simulink model "Problem_8_LIFT"  (R2020b)
settings: Solver=VariableStepAuto  StartTime=0.0  StopTime=10.0  RelTol=1e-3
settings Model: PacingRate=0.450000  Creator=Manoj  LastModifiedBy=Windows 10

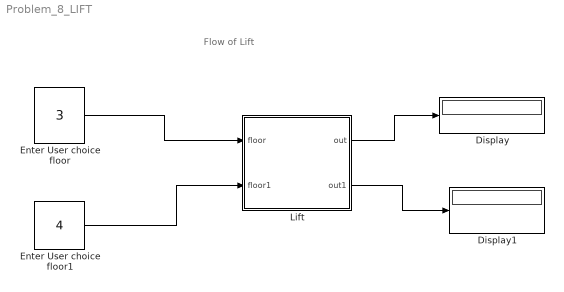
== system Problem_8_LIFT ==
  note: Flow of Lift
  Display : Display
  Display1 : Display
  Enter User choice floor : Constant  Value=3
  Enter User choice floor1 : Constant  Value=4
  Lift : Stateflow chart  TreatAsAtomicUnit=on
  wires:
  Enter User choice floor/1 -> Lift/1(floor)
  Lift/1(out) -> Display/1
  Enter User choice floor1/1 -> Lift/2(floor1)
  Lift/2(out1) -> Display1/1

== stateflow chart Problem_8_LIFT/Lift ==
  state Start
    state Lift_For_five_floor
      state Floor1
        entry:
        present=1;
        out=1;
      state Floor2
        entry:
        out=2;
        present=out;
      state Floor3
        entry:
        out=3;
        present=out;
      state Floor4
        entry:
        out=4;
        present=out;
      state Floor5
        entry:
        out=5;
        present=out
      Start.Lift_For_five_floor.Floor1 -> Start.Lift_For_five_floor.Floor1 [order 2] : [present==floor]
      (default) -> Start.Lift_For_five_floor.Floor1
      Start.Lift_For_five_floor.Floor3 -> Start.Lift_For_five_floor.Floor4 [order 1] : [present<floor]
      Start.Lift_For_five_floor.Floor2 -> Start.Lift_For_five_floor.Floor3 [order 1] : [present<floor]
      Start.Lift_For_five_floor.Floor4 -> Start.Lift_For_five_floor.Floor5 [order 1] : [present<floor]
      Start.Lift_For_five_floor.Floor1 -> Start.Lift_For_five_floor.Floor2 [order 1] : [present<floor]
      Start.Lift_For_five_floor.Floor5 -> Start.Lift_For_five_floor.Floor5 [order 2] : [floor==present]
      Start.Lift_For_five_floor.Floor5 -> Start.Lift_For_five_floor.Floor4 [order 1] : [present>floor]
      Start.Lift_For_five_floor.Floor4 -> Start.Lift_For_five_floor.Floor3 [order 2] : [present>floor]
      Start.Lift_For_five_floor.Floor2 -> Start.Lift_For_five_floor.Floor1 [order 2] : [present>floor]
      Start.Lift_For_five_floor.Floor3 -> Start.Lift_For_five_floor.Floor2 [order 2] : [present>floor]
    state Second_input
      state Floor1
        entry:
        present=1;
        out1=1;
      state Floor2
        entry:
        out1=2;
        present=out1;
      state Floor3
        entry:
        out1=3;
        present=out1;
      state Floor4
        entry:
        out1=4;
        present=out1;
      state Floor5
        entry:
        out1=5;
        present=out1;
      Start.Second_input.Floor1 -> Start.Second_input.Floor1 [order 2] : [present==floor1]
      (default) -> Start.Second_input.Floor1
      Start.Second_input.Floor3 -> Start.Second_input.Floor4 [order 1] : [present<floor1]
      Start.Second_input.Floor2 -> Start.Second_input.Floor3 [order 1] : [present<floor1]
      Start.Second_input.Floor4 -> Start.Second_input.Floor5 [order 1] : [present<floor1]
      Start.Second_input.Floor1 -> Start.Second_input.Floor2 [order 1] : [present<floor1]
      Start.Second_input.Floor5 -> Start.Second_input.Floor5 [order 2] : [floor==present]
      Start.Second_input.Floor5 -> Start.Second_input.Floor4 [order 1] : [present>floor1]
      Start.Second_input.Floor4 -> Start.Second_input.Floor3 [order 2] : [present>floor1]
      Start.Second_input.Floor2 -> Start.Second_input.Floor1 [order 2] : [present>floor1]
      Start.Second_input.Floor3 -> Start.Second_input.Floor2 [order 2] : [present>floor1]
    (default) -> Lift_For_five_floor
    Lift_For_five_floor -> Second_input : [present==floor]
  (default) -> Start
  data: floor input; present local; out output; floor1 input; out1 output
